simulink library "reaction_wheel_assembly_lib_disc"  (R2018b)
settings: Solver=VariableStepAuto  StartTime=0.0  StopTime=10.0  RelTol=1e-3
undefined symbols (not defined in the file): fswParams, simParams
libraries: reaction_wheel_PID_lib x4, rw_motor_lib_disc x4, rw_valid_lib x1
settings Model: Creator=unsik  LastModifiedBy=colem
settings SFSimCC: SimUseLocalCustomCode=off
settings RTWCC: RTWUseLocalCustomCode=off
settings CodeAppCC: StateflowObjectComments=on

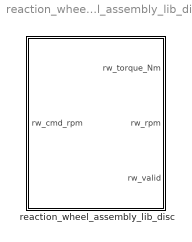
== system reaction_wheel_assembly_lib_disc ==
  reaction_wheel_assembly_lib_disc : Subsystem

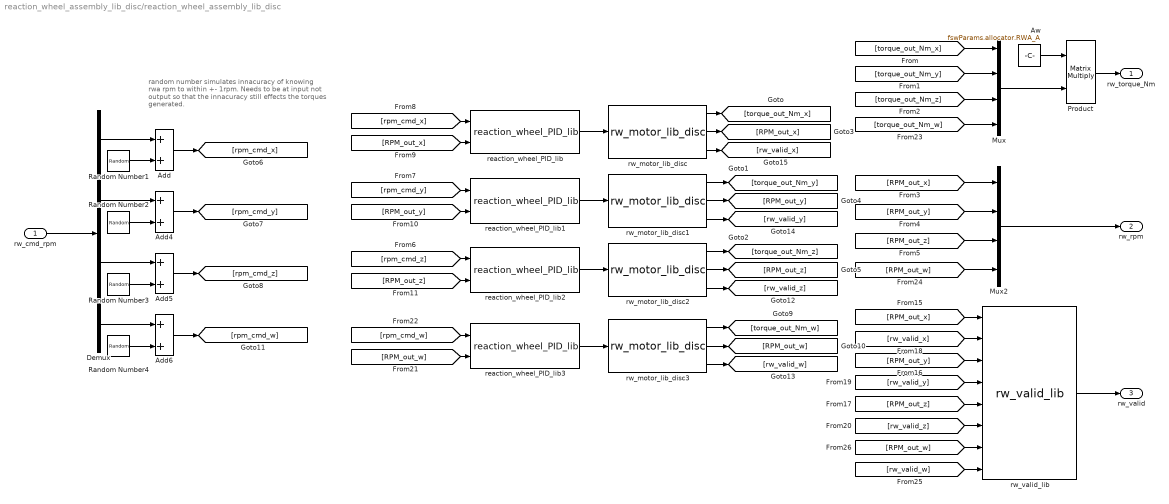
== system reaction_wheel_assembly_lib_disc/reaction_wheel_assembly_lib_disc ==
  note: random number simulates innacuracy of knowing rwa rpm to within +- 1rpm. Needs to be at input not output so that the innacuracy still effects the torques generated.
  rw_cmd_rpm : Inport
  Add{,4..6} (4 alike) : Sum
  Aw : Constant  Value=fswParams.allocator.RWA_A  SampleTime=simParams.sample_time_s
  Demux : Demux
  Mux : Mux
  Mux2 : Mux
  Product : Product  Multiplication=Matrix(*)
  Random Number1 : RandomNumber  Variance=simParams.actuators.rwa.rpm_variance  Seed=1  SampleTime=simParams.sample_time_s
  Random Number2 : RandomNumber  Variance=simParams.actuators.rwa.rpm_variance  Seed=2  SampleTime=simParams.sample_time_s
  Random Number3 : RandomNumber  Variance=simParams.actuators.rwa.rpm_variance  Seed=3  SampleTime=simParams.sample_time_s
  Random Number4 : RandomNumber  Variance=simParams.actuators.rwa.rpm_variance  Seed=4  SampleTime=simParams.sample_time_s
  reaction_wheel_PID_lib{,1..3} (4 alike) : reaction_wheel_PID_lib/reaction_wheel_PID_lib  SystemSampleTime=-1
  rw_motor_lib_disc : rw_motor_lib_disc/rw_motor_lib_disc  id_a=1
  rw_motor_lib_disc1 : rw_motor_lib_disc/rw_motor_lib_disc  id_a=2
  rw_motor_lib_disc2 : rw_motor_lib_disc/rw_motor_lib_disc  id_a=3
  rw_motor_lib_disc3 : rw_motor_lib_disc/rw_motor_lib_disc  id_a=4
  rw_valid_lib : rw_valid_lib/rw_valid_lib  SystemSampleTime=-1
  rw_torque_Nm : Outport
  rw_rpm : Outport  Port=2
  rw_valid : Outport  Port=3
  wires:
  [rw_valid_w] -> rw_valid_lib/8
  [rw_valid_z] -> rw_valid_lib/6
  [rw_valid_y] -> rw_valid_lib/4
  [rw_valid_x] -> rw_valid_lib/2
  [torque_out_Nm_w] -> Mux/4
  rw_motor_lib_disc/3 -> [rw_valid_x]
  rw_motor_lib_disc1/3 -> [rw_valid_y]
  Demux/4 -> Add6/1
  rw_motor_lib_disc3/3 -> [rw_valid_w]
  [RPM_out_w] -> reaction_wheel_PID_lib3/2
  reaction_wheel_PID_lib3/1 -> rw_motor_lib_disc3/1
  rw_motor_lib_disc3/1 -> [torque_out_Nm_w]
  [rpm_cmd_w] -> reaction_wheel_PID_lib3/1
  rw_motor_lib_disc3/2 -> [RPM_out_w]
  rw_motor_lib_disc2/3 -> [rw_valid_z]
  reaction_wheel_PID_lib/1 -> rw_motor_lib_disc/1
  Demux/1 -> Add/1
  reaction_wheel_PID_lib1/1 -> rw_motor_lib_disc1/1
  reaction_wheel_PID_lib2/1 -> rw_motor_lib_disc2/1
  rw_cmd_rpm/1 -> Demux/1
  [torque_out_Nm_x] -> Mux/1
  [torque_out_Nm_y] -> Mux/2
  [torque_out_Nm_z] -> Mux/3
  rw_motor_lib_disc1/2 -> [RPM_out_y]
  rw_motor_lib_disc2/2 -> [RPM_out_z]
  rw_motor_lib_disc/2 -> [RPM_out_x]
  rw_motor_lib_disc/1 -> [torque_out_Nm_x]
  rw_motor_lib_disc2/1 -> [torque_out_Nm_z]
  rw_motor_lib_disc1/1 -> [torque_out_Nm_y]
  [RPM_out_x] -> reaction_wheel_PID_lib/2
  [RPM_out_y] -> reaction_wheel_PID_lib1/2
  [RPM_out_z] -> reaction_wheel_PID_lib2/2
  Product/1 -> rw_torque_Nm/1
  Demux/2 -> Add4/1
  [rpm_cmd_z] -> reaction_wheel_PID_lib2/1
  [rpm_cmd_y] -> reaction_wheel_PID_lib1/1
  [rpm_cmd_x] -> reaction_wheel_PID_lib/1
  rw_valid_lib/1 -> rw_valid/1
  Mux/1 -> Product/2
  Aw/1 -> Product/1
  [RPM_out_z] -> rw_valid_lib/5
  [RPM_out_x] -> rw_valid_lib/1
  [RPM_out_y] -> rw_valid_lib/3
  [RPM_out_w] -> rw_valid_lib/7
  Mux2/1 -> rw_rpm/1
  [RPM_out_x] -> Mux2/1
  Random Number1/1 -> Add/2
  Random Number3/1 -> Add5/2
  Add6/1 -> [rpm_cmd_w]
  [RPM_out_y] -> Mux2/2
  [RPM_out_z] -> Mux2/3
  Random Number4/1 -> Add6/2
  Random Number2/1 -> Add4/2
  Add4/1 -> [rpm_cmd_y]
  Add/1 -> [rpm_cmd_x]
  Add5/1 -> [rpm_cmd_z]
  [RPM_out_w] -> Mux2/4
  Demux/3 -> Add5/1
